simulink model "wheel"  (R2017b)
settings: Solver=VariableStepAuto  StartTime=0.0  StopTime=10.0  RelTol=1e-3
model mask{tyremodel=0}
model workspace (MAT data in the model file):
  tyremodel = 0
settings Model: ParameterArgumentNames=tyremodel  OrderedModelArguments=off  Creator=Seb  LastModifiedBy=Seb

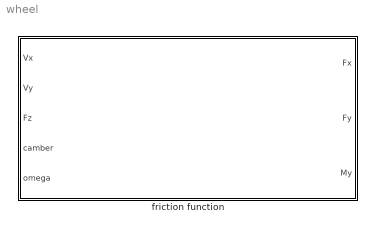
== system wheel ==
  "friction function " : MATLAB Function  TreatAsAtomicUnit=on

== matlab function wheel/friction function  ==
  data: Vx input; Fx output; Vy input; Fz input; camber input; omega input; Fy output; My output
function [Fx, Fy, My] = friction(Vx, Vy, Fz, camber, omega)


end
